simulink model "sfcndemo_io_handling"  (Simulink 6.0)
settings: Solver=ode3  StartTime=0.0  StopTime=10.0  RelTol=1e-3
PreLoadFcn:
  | t=0;u=[1 2 3 4 5 0 0 0 0 0 0 0 0 0 0];
undefined symbols (not defined in the file or in its folder): DiscIntNeverNeededParam
settings Model: CovMetricSettings=d  Creator=The MathWorks Inc.  LastModifiedBy=batserve  ExtModeAutoUpdateStatusClock=off
settings DataIOCC: LoadExternalInput=on  SaveState=on
settings OptimizationCC: BlockReduction=off  BooleanDataType=off  InlineInvariantSignals=off
settings DebuggingCC: ConsistencyChecking=error  CheckExecutionContextPreStartOutputMsg=on  CheckExecutionContextRuntimeOutputMsg=on  SolverPrmCheckMsg=none
settings HardwareCC: TargetUnknown=on
settings RTWCC: RetainRTWFile=on

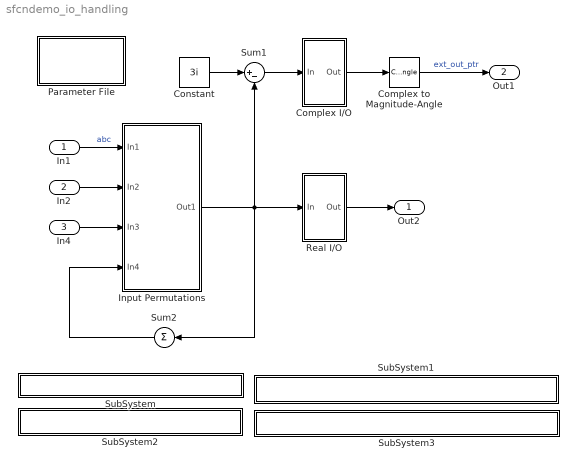
== system sfcndemo_io_handling ==
  In1 : Inport  Port=1  PortDimensions=5  LatchInput=off
  In2 : Inport  Port=2  PortDimensions=5  LatchInput=off
  In4 : Inport  Port=3  PortDimensions=5  LatchInput=off
      settings: SignalType=complex
  Complex I/O : Subsystem  PropExecContextAcrossSSBoundary=on
  Complex to Magnitude-Angle : ComplexToMagnitudeAngle  Output=Magnitude
  Constant : Constant  Value=3i
  Input Permutations : Subsystem  PropExecContextAcrossSSBoundary=on
  Parameter File : Subsystem  PropExecContextAcrossSSBoundary=on
      settings: CopyFcn=cccopyfcn(gcb)  OpenFcn=ccopenfcn('Parameter File')
      mask Type: Parameter File
      mask Description: Add code to model .prm file
      mask Help: This parameter file block contains text fields to insert custom user code at the top and bottom of model.prm file.
      mask Display: disp('Parameter\nFile');
  Real I/O : Subsystem  PropExecContextAcrossSSBoundary=on
  SubSystem : Subsystem  PropExecContextAcrossSSBoundary=on
      settings: OpenFcn=edit(fullfile(matlabroot,'simulink','src','sfun_io_handling1.c'))
      mask Display: disp('matlabroot\simulink\src\sfun_io_handling1.c');
  SubSystem1 : Subsystem  PropExecContextAcrossSSBoundary=on
      settings: OpenFcn=edit(fullfile(matlabroot,'toolbox','simulink','blocks','tlc_c','sfun_io_handling1.tlc'))
      mask Display: disp('matlabroot\toolbox\simulink\blocks\tlc_c\sfun_io_handling1.tlc');
  SubSystem2 : Subsystem  PropExecContextAcrossSSBoundary=on
      settings: OpenFcn=edit(fullfile(matlabroot,'simulink','src','sfun_io_handling2.c'))
      mask Display: disp('matlabroot\simulink\src\sfun_io_handling2.c');
  SubSystem3 : Subsystem  PropExecContextAcrossSSBoundary=on
      settings: OpenFcn=edit(fullfile(matlabroot,'toolbox','simulink','blocks','tlc_c','sfun_io_handling2.tlc'))
      mask Display: disp('matlabroot\toolbox\simulink\blocks\tlc_c\sfun_io_handling2.tlc');
  Sum1 : Sum  Inputs=|+-  SaturateOnIntegerOverflow=on  InputSameDT=on
  Sum2 : Sum  Orientation=left  Inputs=+  SaturateOnIntegerOverflow=on  InputSameDT=on
  Out2 : Outport
  Out1 : Outport  Port=2
  wires:
  In1/1 -> Input Permutations/1(In1)  "abc"
  In4/1 -> Input Permutations/3(In3)
  Sum2/1 -> Input Permutations/4(In4)
  Complex I/O/1(Out) -> Complex to Magnitude-Angle/1
  In2/1 -> Input Permutations/2(In2)
  Input Permutations/1(Out1) -> Real I/O/1(In), Sum2/1, Sum1/2
  Real I/O/1(Out) -> Out2/1
  Complex to Magnitude-Angle/1 -> Out1/1  "ext_out_ptr"
  Sum1/1 -> Complex I/O/1(In)
  Constant/1 -> Sum1/1

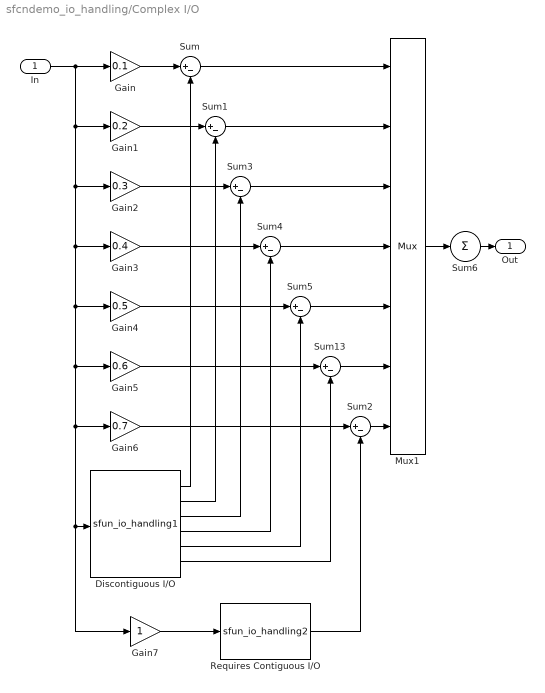
== system sfcndemo_io_handling/Complex I/O ==
  In : Inport  Port=1  LatchInput=off
  Discontiguous I/O : S-Function  FunctionName=sfun_io_handling1
  Gain : Gain  Gain=0.1  SaturateOnIntegerOverflow=on
  Gain1 : Gain  Gain=0.2  SaturateOnIntegerOverflow=on
  Gain2 : Gain  Gain=0.3  SaturateOnIntegerOverflow=on
  Gain3 : Gain  Gain=0.4  SaturateOnIntegerOverflow=on
  Gain4 : Gain  Gain=0.5  SaturateOnIntegerOverflow=on
  Gain5 : Gain  Gain=0.6  SaturateOnIntegerOverflow=on
  Gain6 : Gain  Gain=0.7  SaturateOnIntegerOverflow=on
  Gain7 : Gain  SaturateOnIntegerOverflow=on
  Mux1 : Mux  Inputs=7
  Requires Contiguous I/O : S-Function  FunctionName=sfun_io_handling2
  Sum{,1..5,13} (7 alike) : Sum  Inputs=|+-  SaturateOnIntegerOverflow=on  InputSameDT=on
  Sum6 : Sum  Inputs=+  SaturateOnIntegerOverflow=on  InputSameDT=on
  Out : Outport
  wires:
  Gain7/1 -> Requires Contiguous I/O/1
  Requires Contiguous I/O/1 -> Sum2/2
  Sum2/1 -> Mux1/7
  Gain6/1 -> Sum2/1
  In/1 -> Gain6/1, Gain7/1, Discontiguous I/O/1, Gain5/1, Gain4/1, Gain3/1, Gain2/1, Gain1/1, Gain/1
  Discontiguous I/O/6 -> Sum13/2
  Gain5/1 -> Sum13/1
  Sum13/1 -> Mux1/6
  Mux1/1 -> Sum6/1
  Sum5/1 -> Mux1/5
  Sum4/1 -> Mux1/4
  Sum3/1 -> Mux1/3
  Sum1/1 -> Mux1/2
  Sum/1 -> Mux1/1
  Sum6/1 -> Out/1
  Discontiguous I/O/5 -> Sum5/2
  Discontiguous I/O/4 -> Sum4/2
  Gain4/1 -> Sum5/1
  Gain3/1 -> Sum4/1
  Discontiguous I/O/3 -> Sum3/2
  Gain2/1 -> Sum3/1
  Discontiguous I/O/2 -> Sum1/2
  Discontiguous I/O/1 -> Sum/2
  Gain1/1 -> Sum1/1
  Gain/1 -> Sum/1

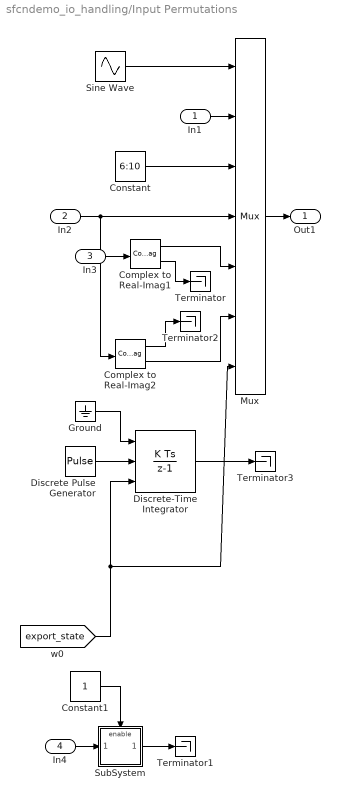
== system sfcndemo_io_handling/Input Permutations ==
  In1 : Inport  Port=1  LatchInput=off
  In2 : Inport  Port=2  LatchInput=off
  In3 : Inport  Port=3  LatchInput=off
  In4 : Inport  Port=4  LatchInput=off
  Complex to Real-Imag1 : ComplexToRealImag
  Complex to Real-Imag2 : ComplexToRealImag
  Constant : Constant  Value=6:10
  Constant1 : Constant
  Discrete Pulse Generator : DiscretePulseGenerator
  Discrete-Time Integrator : DiscreteIntegrator  ExternalReset=either  InitialConditionSource=external  InitialCondition=-5:-1  ICPrevOutput=DiscIntNeverNeededParam  ICPrevScaledInput=DiscIntNeverNeededParam
  Ground : Ground
  Mux : Mux  Inputs=7
  Sine Wave : Sin  Amplitude=1:5  SampleTime=0
  SubSystem : Subsystem  TreatAsAtomicUnit=on  PropExecContextAcrossSSBoundary=on
  Terminator{,1..3} (4 alike) : Terminator
  Out1 : Outport
  wires:
  Sine Wave/1 -> Mux/1
  Constant/1 -> Mux/3
  Constant1/1 -> SubSystem/Enable
  [export_state] -> Discrete-Time Integrator/3, Mux/7
  Discrete Pulse Generator/1 -> Discrete-Time Integrator/2
  Complex to Real-Imag1/1 -> Mux/5
  Complex to Real-Imag2/2 -> Mux/6
  SubSystem/1(Out1) -> Terminator1/1
  Complex to Real-Imag1/2 -> Terminator/1
  Complex to Real-Imag2/1 -> Terminator2/1
  Ground/1 -> Discrete-Time Integrator/1
  Discrete-Time Integrator/1 -> Terminator3/1
  In1/1 -> Mux/2
  In2/1 -> Mux/4, Complex to Real-Imag2/1
  Mux/1 -> Out1/1
  In3/1 -> Complex to Real-Imag1/1
  In4/1 -> SubSystem/1(In1)

== system sfcndemo_io_handling/Parameter File ==

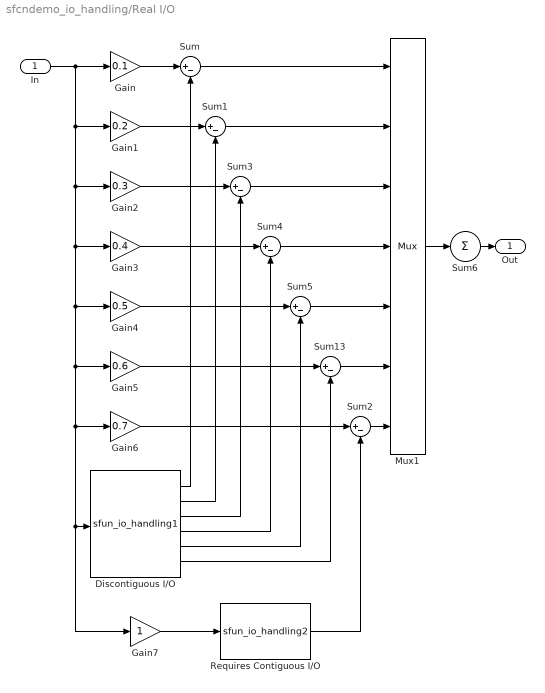
== system sfcndemo_io_handling/Real I/O ==
  In : Inport  Port=1  LatchInput=off
  Discontiguous I/O : S-Function  FunctionName=sfun_io_handling1
  Gain : Gain  Gain=0.1  SaturateOnIntegerOverflow=on
  Gain1 : Gain  Gain=0.2  SaturateOnIntegerOverflow=on
  Gain2 : Gain  Gain=0.3  SaturateOnIntegerOverflow=on
  Gain3 : Gain  Gain=0.4  SaturateOnIntegerOverflow=on
  Gain4 : Gain  Gain=0.5  SaturateOnIntegerOverflow=on
  Gain5 : Gain  Gain=0.6  SaturateOnIntegerOverflow=on
  Gain6 : Gain  Gain=0.7  SaturateOnIntegerOverflow=on
  Gain7 : Gain  SaturateOnIntegerOverflow=on
  Mux1 : Mux  Inputs=7
  Requires Contiguous I/O : S-Function  FunctionName=sfun_io_handling2
  Sum{,1..5,13} (7 alike) : Sum  Inputs=|+-  SaturateOnIntegerOverflow=on  InputSameDT=on
  Sum6 : Sum  Inputs=+  SaturateOnIntegerOverflow=on  InputSameDT=on
  Out : Outport
  wires:
  Gain/1 -> Sum/1
  Gain1/1 -> Sum1/1
  Discontiguous I/O/1 -> Sum/2
  Discontiguous I/O/2 -> Sum1/2
  Gain2/1 -> Sum3/1
  Discontiguous I/O/3 -> Sum3/2
  Gain3/1 -> Sum4/1
  Gain4/1 -> Sum5/1
  Discontiguous I/O/4 -> Sum4/2
  Discontiguous I/O/5 -> Sum5/2
  Sum6/1 -> Out/1
  Sum/1 -> Mux1/1
  Sum1/1 -> Mux1/2
  Sum3/1 -> Mux1/3
  Sum4/1 -> Mux1/4
  Sum5/1 -> Mux1/5
  Mux1/1 -> Sum6/1
  Sum13/1 -> Mux1/6
  Gain5/1 -> Sum13/1
  Discontiguous I/O/6 -> Sum13/2
  In/1 -> Gain/1, Gain1/1, Gain2/1, Gain3/1, Gain4/1, Gain5/1, Discontiguous I/O/1, Gain7/1, Gain6/1
  Gain6/1 -> Sum2/1
  Sum2/1 -> Mux1/7
  Requires Contiguous I/O/1 -> Sum2/2
  Gain7/1 -> Requires Contiguous I/O/1

== system sfcndemo_io_handling/SubSystem ==

== system sfcndemo_io_handling/SubSystem1 ==

== system sfcndemo_io_handling/SubSystem2 ==

== system sfcndemo_io_handling/SubSystem3 ==

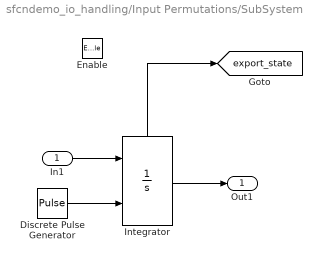
== system sfcndemo_io_handling/Input Permutations/SubSystem ==
  In1 : Inport  Port=1  LatchInput=off
  Enable : EnablePort
  Discrete Pulse Generator : DiscretePulseGenerator
  Integrator : Integrator  ExternalReset=either  InitialCondition=-5:-1  ShowStatePort=on
  Out1 : Outport
  tag scope: export_state=global
  wires:
  In1/1 -> Integrator/1
  Discrete Pulse Generator/1 -> Integrator/2
  Integrator/1 -> Out1/1
  Integrator/State -> [export_state]
